simulink model "case2"  (R2024b)
settings: Solver=FixedStepAuto  StartTime=0  StopTime=1  FixedStep=1e-7  RelTol=1e-3
values from neighbouring files (symbols this model uses):
  SG_D_1_D = 0.01056    [IEEE9_case_parameters.m]    (also in case1_parameters.m; case2_parameters.m; case3_parameters.m; case4_parameters.m)
  SG_D_1_EnableSaturation = 0    [IEEE9_case_parameters.m]    (also in case1_parameters.m; case2_parameters.m; case3_parameters.m; case4_parameters.m)
  SG_D_1_f0 = 60    [IEEE9_case_parameters.m]    (also in case1_parameters.m; case2_parameters.m; case3_parameters.m; case4_parameters.m)
  SG_D_1_H = 7.5    [IEEE9_case_parameters.m]    (also in case1_parameters.m; case2_parameters.m; case3_parameters.m; case4_parameters.m)
  SG_D_1_K_A = 20    [IEEE9_case_parameters.m]    (also in case1_parameters.m; case2_parameters.m; case3_parameters.m; case4_parameters.m)
  SG_D_1_K_E = 1.000000e+1    (= 10)    [IEEE9_case_parameters.m]    (also in case1_parameters.m; case2_parameters.m; case3_parameters.m; case4_parameters.m)
  SG_D_1_K_F = 2.363    [IEEE9_case_parameters.m]    (also in case1_parameters.m; case2_parameters.m; case3_parameters.m; case4_parameters.m)
  SG_D_1_K_s = 0.5    [IEEE9_case_parameters.m]    (also in case1_parameters.m = 5; case2_parameters.m = 5; case3_parameters.m = 5; case4_parameters.m = 5)
  SG_D_1_R_a = 0.001088    [IEEE9_case_parameters.m]    (also in case1_parameters.m; case2_parameters.m; case3_parameters.m; case4_parameters.m)
  SG_D_1_S_A = 1    [IEEE9_case_parameters.m]    (also in case1_parameters.m; case2_parameters.m; case3_parameters.m; case4_parameters.m)
  SG_D_1_S_B = 0.103    [IEEE9_case_parameters.m]    (also in case1_parameters.m; case2_parameters.m; case3_parameters.m; case4_parameters.m)
  SG_D_1_S_N = 10.659857    [IEEE9_case_parameters.m]    (also in case1_parameters.m; case2_parameters.m; case3_parameters.m; case4_parameters.m)
  SG_D_1_SpeedPara = 200    [IEEE9_case_parameters.m]    (also in case1_parameters.m; case2_parameters.m; case3_parameters.m; case4_parameters.m)
  SG_D_1_T_0 = 0.720173    [IEEE9_case_parameters.m]    (also in case1_parameters.m = 0.755522; case2_parameters.m = 0.808931; case3_parameters.m = 0.869402; case4_parameters.m = 0.729316)
  SG_D_1_T_1 = 0.3    [IEEE9_case_parameters.m]    (also in case1_parameters.m; case2_parameters.m; case3_parameters.m; case4_parameters.m)
  SG_D_1_T_2 = 0.05    [IEEE9_case_parameters.m]    (also in case1_parameters.m; case2_parameters.m; case3_parameters.m; case4_parameters.m)
  SG_D_1_T_3 = 0.02    [IEEE9_case_parameters.m]    (also in case1_parameters.m; case2_parameters.m; case3_parameters.m; case4_parameters.m)
  SG_D_1_T_4 = 0.005    [IEEE9_case_parameters.m]    (also in case1_parameters.m; case2_parameters.m; case3_parameters.m; case4_parameters.m)
  SG_D_1_T_A = 0.02    [IEEE9_case_parameters.m]    (also in case1_parameters.m; case2_parameters.m; case3_parameters.m; case4_parameters.m)
  SG_D_1_T_dd = 8.000000e+0    (= 8)    [IEEE9_case_parameters.m]    (also in case1_parameters.m; case2_parameters.m; case3_parameters.m; case4_parameters.m)
  SG_D_1_T_ddd = 0.04    [IEEE9_case_parameters.m]    (also in case1_parameters.m; case2_parameters.m; case3_parameters.m; case4_parameters.m)
  SG_D_1_T_E = 0.314    [IEEE9_case_parameters.m]    (also in case1_parameters.m; case2_parameters.m; case3_parameters.m; case4_parameters.m)
  SG_D_1_T_F = 0.35    [IEEE9_case_parameters.m]    (also in case1_parameters.m; case2_parameters.m; case3_parameters.m; case4_parameters.m)
  SG_D_1_T_qd = 0.8    [IEEE9_case_parameters.m]    (also in case1_parameters.m; case2_parameters.m; case3_parameters.m; case4_parameters.m)
  SG_D_1_T_qdd = 0.02    [IEEE9_case_parameters.m]    (also in case1_parameters.m; case2_parameters.m; case3_parameters.m; case4_parameters.m)
  SG_D_1_T_speed = 0.1    [IEEE9_case_parameters.m]    (also in case1_parameters.m = 200; case2_parameters.m = 200; case3_parameters.m = 200; case4_parameters.m = 200)
  SG_D_1_T_w = 0.5    [IEEE9_case_parameters.m]    (also in case1_parameters.m; case2_parameters.m; case3_parameters.m; case4_parameters.m)
  SG_D_1_V_ref = 1.990276    [IEEE9_case_parameters.m]    (also in case1_parameters.m = 2.042296; case2_parameters.m = 2.051388; case3_parameters.m = 2.089584; case4_parameters.m = 2.01845)
  SG_D_1_w_ref = 376.991118    [IEEE9_case_parameters.m]    (also in case1_parameters.m; case2_parameters.m; case3_parameters.m; case4_parameters.m)
  SG_D_1_wb = 6.000000e+1    (= 60)    [IEEE9_case_parameters.m]    (also in case1_parameters.m; case2_parameters.m; case3_parameters.m; case4_parameters.m)
  SG_D_1_x_d = 1.9    [IEEE9_case_parameters.m]    (also in case1_parameters.m; case2_parameters.m; case3_parameters.m; case4_parameters.m)
  SG_D_1_x_dd = 0.302    [IEEE9_case_parameters.m]    (also in case1_parameters.m; case2_parameters.m; case3_parameters.m; case4_parameters.m)
  SG_D_1_x_ddd = 0.204    [IEEE9_case_parameters.m]    (also in case1_parameters.m; case2_parameters.m; case3_parameters.m; case4_parameters.m)
  SG_D_1_x_l = 0.05    [IEEE9_case_parameters.m]    (also in case1_parameters.m; case2_parameters.m; case3_parameters.m; case4_parameters.m)
  SG_D_1_x_q = 1.3    [IEEE9_case_parameters.m]    (also in case1_parameters.m; case2_parameters.m; case3_parameters.m; case4_parameters.m)
  SG_D_1_x_qd = 0.5    [IEEE9_case_parameters.m]    (also in case1_parameters.m; case2_parameters.m; case3_parameters.m; case4_parameters.m)
  SG_D_1_x_qdd = 0.3    [IEEE9_case_parameters.m]    (also in case1_parameters.m; case2_parameters.m; case3_parameters.m; case4_parameters.m)
  SG_D_2_D = 0.02    [IEEE9_case_parameters.m]    (also in case1_parameters.m; case2_parameters.m; case3_parameters.m; case4_parameters.m)
  SG_D_2_EnableSaturation = 0    [IEEE9_case_parameters.m]    (also in case1_parameters.m; case2_parameters.m; case3_parameters.m; case4_parameters.m)
  SG_D_2_f0 = 60    [IEEE9_case_parameters.m]    (also in case1_parameters.m; case2_parameters.m; case3_parameters.m; case4_parameters.m)
  SG_D_2_H = 8.000000e+0    (= 8)    [IEEE9_case_parameters.m]    (also in case1_parameters.m; case2_parameters.m; case3_parameters.m; case4_parameters.m)
  SG_D_2_K_A = 20    [IEEE9_case_parameters.m]    (also in case1_parameters.m; case2_parameters.m; case3_parameters.m; case4_parameters.m)
  SG_D_2_K_E = 1.000000e+1    (= 10)    [IEEE9_case_parameters.m]    (also in case1_parameters.m; case2_parameters.m; case3_parameters.m; case4_parameters.m)
  SG_D_2_K_F = 2.363    [IEEE9_case_parameters.m]    (also in case1_parameters.m; case2_parameters.m; case3_parameters.m; case4_parameters.m)
  SG_D_2_K_s = 0.5    [IEEE9_case_parameters.m]    (also in case1_parameters.m = 4; case2_parameters.m = 4; case3_parameters.m = 4; case4_parameters.m = 4)
  SG_D_2_R_a = 0.001088    [IEEE9_case_parameters.m]    (also in case1_parameters.m; case2_parameters.m; case3_parameters.m; case4_parameters.m)
  SG_D_2_S_A = 1    [IEEE9_case_parameters.m]    (also in case1_parameters.m; case2_parameters.m; case3_parameters.m; case4_parameters.m)
  SG_D_2_S_B = 0.103    [IEEE9_case_parameters.m]    (also in case1_parameters.m; case2_parameters.m; case3_parameters.m; case4_parameters.m)
  SG_D_2_S_N = 10.659857    [IEEE9_case_parameters.m]    (also in case1_parameters.m; case2_parameters.m; case3_parameters.m; case4_parameters.m)
  SG_D_2_SpeedPara = 200    [IEEE9_case_parameters.m]    (also in case1_parameters.m; case2_parameters.m; case3_parameters.m; case4_parameters.m)
  SG_D_2_T_0 = 1.632913    [IEEE9_case_parameters.m]    (also in case1_parameters.m = 1.632925; case2_parameters.m = 1.632915; case3_parameters.m = 1.632914; case4_parameters.m = 1.632927)
  SG_D_2_T_1 = 0.2    [IEEE9_case_parameters.m]    (also in case1_parameters.m; case2_parameters.m; case3_parameters.m; case4_parameters.m)
  SG_D_2_T_2 = 0.05    [IEEE9_case_parameters.m]    (also in case1_parameters.m; case2_parameters.m; case3_parameters.m; case4_parameters.m)
  SG_D_2_T_3 = 0.02    [IEEE9_case_parameters.m]    (also in case1_parameters.m; case2_parameters.m; case3_parameters.m; case4_parameters.m)
  SG_D_2_T_4 = 0.005    [IEEE9_case_parameters.m]    (also in case1_parameters.m; case2_parameters.m; case3_parameters.m; case4_parameters.m)
  SG_D_2_T_A = 0.02    [IEEE9_case_parameters.m]    (also in case1_parameters.m; case2_parameters.m; case3_parameters.m; case4_parameters.m)
  SG_D_2_T_dd = 7.9    [IEEE9_case_parameters.m]    (also in case1_parameters.m; case2_parameters.m; case3_parameters.m; case4_parameters.m)
  SG_D_2_T_ddd = 0.04    [IEEE9_case_parameters.m]    (also in case1_parameters.m; case2_parameters.m; case3_parameters.m; case4_parameters.m)
  SG_D_2_T_E = 0.314    [IEEE9_case_parameters.m]    (also in case1_parameters.m; case2_parameters.m; case3_parameters.m; case4_parameters.m)
  SG_D_2_T_F = 0.35    [IEEE9_case_parameters.m]    (also in case1_parameters.m; case2_parameters.m; case3_parameters.m; case4_parameters.m)
  SG_D_2_T_qd = 0.8    [IEEE9_case_parameters.m]    (also in case1_parameters.m; case2_parameters.m; case3_parameters.m; case4_parameters.m)
  SG_D_2_T_qdd = 0.015    [IEEE9_case_parameters.m]    (also in case1_parameters.m; case2_parameters.m; case3_parameters.m; case4_parameters.m)
  SG_D_2_T_speed = 0.1    [IEEE9_case_parameters.m]    (also in case1_parameters.m = 150; case2_parameters.m = 150; case3_parameters.m = 150; case4_parameters.m = 150)
  SG_D_2_T_w = 0.35    [IEEE9_case_parameters.m]    (also in case1_parameters.m; case2_parameters.m; case3_parameters.m; case4_parameters.m)
  SG_D_2_V_ref = 2.58547    [IEEE9_case_parameters.m]    (also in case1_parameters.m = 2.597896; case2_parameters.m = 2.587136; case3_parameters.m = 2.586042; case4_parameters.m = 2.599679)
  SG_D_2_w_ref = 376.991118    [IEEE9_case_parameters.m]    (also in case1_parameters.m; case2_parameters.m; case3_parameters.m; case4_parameters.m)
  SG_D_2_wb = 6.000000e+1    (= 60)    [IEEE9_case_parameters.m]    (also in case1_parameters.m; case2_parameters.m; case3_parameters.m; case4_parameters.m)
  SG_D_2_x_d = 1.8    [IEEE9_case_parameters.m]    (also in case1_parameters.m; case2_parameters.m; case3_parameters.m; case4_parameters.m)
  SG_D_2_x_dd = 0.302    [IEEE9_case_parameters.m]    (also in case1_parameters.m; case2_parameters.m; case3_parameters.m; case4_parameters.m)
  SG_D_2_x_ddd = 0.204    [IEEE9_case_parameters.m]    (also in case1_parameters.m; case2_parameters.m; case3_parameters.m; case4_parameters.m)
  SG_D_2_x_l = 0.05    [IEEE9_case_parameters.m]    (also in case1_parameters.m; case2_parameters.m; case3_parameters.m; case4_parameters.m)
  SG_D_2_x_q = 1.25    [IEEE9_case_parameters.m]    (also in case1_parameters.m; case2_parameters.m; case3_parameters.m; case4_parameters.m)
  SG_D_2_x_qd = 0.5    [IEEE9_case_parameters.m]    (also in case1_parameters.m; case2_parameters.m; case3_parameters.m; case4_parameters.m)
  SG_D_2_x_qdd = 0.3    [IEEE9_case_parameters.m]    (also in case1_parameters.m; case2_parameters.m; case3_parameters.m; case4_parameters.m)
  SG_D_3_D = 0.02    [IEEE9_case_parameters.m]    (also in case1_parameters.m; case2_parameters.m; case3_parameters.m; case4_parameters.m)
  SG_D_3_EnableSaturation = 0    [IEEE9_case_parameters.m]    (also in case1_parameters.m; case2_parameters.m; case3_parameters.m; case4_parameters.m)
  SG_D_3_f0 = 60    [IEEE9_case_parameters.m]    (also in case1_parameters.m; case2_parameters.m; case3_parameters.m; case4_parameters.m)
  SG_D_3_H = 7.7    [IEEE9_case_parameters.m]    (also in case1_parameters.m; case2_parameters.m; case3_parameters.m; case4_parameters.m)
  SG_D_3_K_A = 20    [IEEE9_case_parameters.m]    (also in case1_parameters.m; case2_parameters.m; case3_parameters.m; case4_parameters.m)
  SG_D_3_K_E = 1.000000e+1    (= 10)    [IEEE9_case_parameters.m]    (also in case1_parameters.m; case2_parameters.m; case3_parameters.m; case4_parameters.m)
  SG_D_3_K_F = 2.363    [IEEE9_case_parameters.m]    (also in case1_parameters.m; case2_parameters.m; case3_parameters.m; case4_parameters.m)
  SG_D_3_K_s = 0.2    [IEEE9_case_parameters.m]    (also in case1_parameters.m = 2; case2_parameters.m = 2; case3_parameters.m = 2; case4_parameters.m = 2)
  SG_D_3_R_a = 0.001088    [IEEE9_case_parameters.m]    (also in case1_parameters.m; case2_parameters.m; case3_parameters.m; case4_parameters.m)
  SG_D_3_S_A = 1    [IEEE9_case_parameters.m]    (also in case1_parameters.m; case2_parameters.m; case3_parameters.m; case4_parameters.m)
  SG_D_3_S_B = 0.103    [IEEE9_case_parameters.m]    (also in case1_parameters.m; case2_parameters.m; case3_parameters.m; case4_parameters.m)
  SG_D_3_S_N = 10.659857    [IEEE9_case_parameters.m]    (also in case1_parameters.m; case2_parameters.m; case3_parameters.m; case4_parameters.m)
  SG_D_3_SpeedPara = 200    [IEEE9_case_parameters.m]    (also in case1_parameters.m; case2_parameters.m; case3_parameters.m; case4_parameters.m)
  SG_D_3_T_0 = 0.850788    [IEEE9_case_parameters.m]    (also in case1_parameters.m = 0.850786; case2_parameters.m = 0.850787; case3_parameters.m; case4_parameters.m = 0.850786)
  SG_D_3_T_1 = 0.2    [IEEE9_case_parameters.m]    (also in case1_parameters.m; case2_parameters.m; case3_parameters.m; case4_parameters.m)
  SG_D_3_T_2 = 0.05    [IEEE9_case_parameters.m]    (also in case1_parameters.m; case2_parameters.m; case3_parameters.m; case4_parameters.m)
  SG_D_3_T_3 = 0.02    [IEEE9_case_parameters.m]    (also in case1_parameters.m; case2_parameters.m; case3_parameters.m; case4_parameters.m)
  SG_D_3_T_4 = 0.005    [IEEE9_case_parameters.m]    (also in case1_parameters.m; case2_parameters.m; case3_parameters.m; case4_parameters.m)
  SG_D_3_T_A = 0.02    [IEEE9_case_parameters.m]    (also in case1_parameters.m; case2_parameters.m; case3_parameters.m; case4_parameters.m)
  SG_D_3_T_dd = 8.1    [IEEE9_case_parameters.m]    (also in case1_parameters.m; case2_parameters.m; case3_parameters.m; case4_parameters.m)
  SG_D_3_T_ddd = 0.04    [IEEE9_case_parameters.m]    (also in case1_parameters.m; case2_parameters.m; case3_parameters.m; case4_parameters.m)
  SG_D_3_T_E = 0.314    [IEEE9_case_parameters.m]    (also in case1_parameters.m; case2_parameters.m; case3_parameters.m; case4_parameters.m)
  SG_D_3_T_F = 0.35    [IEEE9_case_parameters.m]    (also in case1_parameters.m; case2_parameters.m; case3_parameters.m; case4_parameters.m)
  SG_D_3_T_qd = 0.8    [IEEE9_case_parameters.m]    (also in case1_parameters.m; case2_parameters.m; case3_parameters.m; case4_parameters.m)
  SG_D_3_T_qdd = 0.015    [IEEE9_case_parameters.m]    (also in case1_parameters.m; case2_parameters.m; case3_parameters.m; case4_parameters.m)
  SG_D_3_T_speed = 0.1    [IEEE9_case_parameters.m]    (also in case1_parameters.m = 180; case2_parameters.m = 180; case3_parameters.m = 180; case4_parameters.m = 180)
  SG_D_3_T_w = 0.4    [IEEE9_case_parameters.m]    (also in case1_parameters.m; case2_parameters.m; case3_parameters.m; case4_parameters.m)
  SG_D_3_V_ref = 1.892727    [IEEE9_case_parameters.m]    (also in case1_parameters.m = 1.906439; case2_parameters.m = 1.895535; case3_parameters.m = 1.892105; case4_parameters.m = 1.906598)
  SG_D_3_w_ref = 376.991118    [IEEE9_case_parameters.m]    (also in case1_parameters.m; case2_parameters.m; case3_parameters.m; case4_parameters.m)
  SG_D_3_wb = 6.000000e+1    (= 60)    [IEEE9_case_parameters.m]    (also in case1_parameters.m; case2_parameters.m; case3_parameters.m; case4_parameters.m)
  SG_D_3_x_d = 1.85    [IEEE9_case_parameters.m]    (also in case1_parameters.m; case2_parameters.m; case3_parameters.m; case4_parameters.m)
  SG_D_3_x_dd = 0.302    [IEEE9_case_parameters.m]    (also in case1_parameters.m; case2_parameters.m; case3_parameters.m; case4_parameters.m)
  SG_D_3_x_ddd = 0.204    [IEEE9_case_parameters.m]    (also in case1_parameters.m; case2_parameters.m; case3_parameters.m; case4_parameters.m)
  SG_D_3_x_l = 0.05    [IEEE9_case_parameters.m]    (also in case1_parameters.m; case2_parameters.m; case3_parameters.m; case4_parameters.m)
  SG_D_3_x_q = 1.2    [IEEE9_case_parameters.m]    (also in case1_parameters.m; case2_parameters.m; case3_parameters.m; case4_parameters.m)
  SG_D_3_x_qd = 0.5    [IEEE9_case_parameters.m]    (also in case1_parameters.m; case2_parameters.m; case3_parameters.m; case4_parameters.m)
  SG_D_3_x_qdd = 0.3    [IEEE9_case_parameters.m]    (also in case1_parameters.m; case2_parameters.m; case3_parameters.m; case4_parameters.m)
(part 3 of 12)

== system case2/AC_1/d_id_load_7_block ==
  note: d_id_load_7 in case2
      | $376.991118430775\,\mathrm{iq}_{\mathrm{load},7}-1094.41926714385\,\mathrm{id}_{\mathrm{load},7}+1297.48703148083\,\mathrm{vd}_{\mathrm{bus},7}$
      | Automatically generated on 2025-10-31 18:56:46 .
  State_id_load_7_50270 : Inport
  State_iq_load_7_f0642 : Inport  Port=2
  State_vd_bus_7_8233e : Inport  Port=3
  Add_35670 : Sum
  Add_ebaa6 : Sum
  Constant_-1094.41926714385_6f1bd : Constant  Value=-1094.41926714385
  Constant_1297.48703148083_7e1ab : Constant  Value=1297.48703148083
  Constant_376.991118430775_2a44c : Constant  Value=376.991118430775
  Product_56fc3 : Product
  Product_c3dd4 : Product
  Product_fbb26 : Product
  Blockout_d_id_load_7_5a75a : Outport
  wires:
  Constant_-1094.41926714385_6f1bd/1 -> Product_56fc3/1
  Product_fbb26/1 -> Add_ebaa6/2
  State_id_load_7_50270/1 -> Product_56fc3/2
  Constant_376.991118430775_2a44c/1 -> Product_fbb26/1
  Product_56fc3/1 -> Add_ebaa6/1
  State_iq_load_7_f0642/1 -> Product_fbb26/2
  Constant_1297.48703148083_7e1ab/1 -> Product_c3dd4/1
  State_vd_bus_7_8233e/1 -> Product_c3dd4/2
  Add_ebaa6/1 -> Add_35670/1
  Product_c3dd4/1 -> Add_35670/2
  Add_35670/1 -> Blockout_d_id_load_7_5a75a/1

== system case2/AC_1/d_id_load_9_block ==
  note: d_id_load_9 in case2
      | $376.991118430775\,\mathrm{iq}_{\mathrm{load},9}-957.616858632595\,\mathrm{id}_{\mathrm{load},9}+1549.09705910486\,\mathrm{vd}_{\mathrm{bus},9}$
      | Automatically generated on 2025-10-31 18:56:48 .
  State_id_load_9_4df15 : Inport
  State_iq_load_9_81910 : Inport  Port=2
  State_vd_bus_9_f0529 : Inport  Port=3
  Add_4a38f : Sum
  Add_6215e : Sum
  Constant_-957.616858632595_0e708 : Constant  Value=-957.616858632595
  Constant_1549.09705910486_dd334 : Constant  Value=1549.09705910486
  Constant_376.991118430775_a5bfc : Constant  Value=376.991118430775
  Product_47c36 : Product
  Product_61caa : Product
  Product_d12cf : Product
  Blockout_d_id_load_9_4d2d3 : Outport
  wires:
  Constant_-957.616858632595_0e708/1 -> Product_47c36/1
  Product_61caa/1 -> Add_4a38f/2
  State_id_load_9_4df15/1 -> Product_47c36/2
  Constant_376.991118430775_a5bfc/1 -> Product_61caa/1
  Product_47c36/1 -> Add_4a38f/1
  State_iq_load_9_81910/1 -> Product_61caa/2
  Constant_1549.09705910486_dd334/1 -> Product_d12cf/1
  State_vd_bus_9_f0529/1 -> Product_d12cf/2
  Add_4a38f/1 -> Add_6215e/1
  Product_d12cf/1 -> Add_6215e/2
  Add_6215e/1 -> Blockout_d_id_load_9_4d2d3/1

== system case2/AC_1/d_iq_line_1_4_block ==
  note: d_iq_line_1_4 in case2
      | $6679.98156752849\,\mathrm{vq}_{\mathrm{bus},1}-376.991118430775\,\mathrm{id}_{\mathrm{line},1,4}-6679.98156752849\,\mathrm{vq}_{\mathrm{bus},4}$
      | Automatically generated on 2025-10-31 18:56:51 .
  State_id_line_1_4_24448 : Inport
  State_vq_bus_1_ed792 : Inport  Port=2
  State_vq_bus_4_1e5cd : Inport  Port=3
  Add_3527d : Sum
  Constant_-376.991118430775_76f6f : Constant  Value=-376.991118430775
  Constant_6679.98156752849_7c1df : Constant  Value=6679.98156752849
  Constant_6679.98156752849_cc398 : Constant  Value=6679.98156752849
  Product_18bbc : Product
  Product_34f2a : Product
  Product_e2593 : Product
  Subtract_9104e : Sum  Inputs=+-
  Blockout_d_iq_line_1_4_76297 : Outport
  wires:
  Constant_-376.991118430775_76f6f/1 -> Product_34f2a/1
  Product_18bbc/1 -> Add_3527d/2
  State_id_line_1_4_24448/1 -> Product_34f2a/2
  Constant_6679.98156752849_cc398/1 -> Product_18bbc/1
  Product_34f2a/1 -> Add_3527d/1
  Subtract_9104e/1 -> Blockout_d_iq_line_1_4_76297/1
  State_vq_bus_1_ed792/1 -> Product_18bbc/2
  Constant_6679.98156752849_7c1df/1 -> Product_e2593/1
  State_vq_bus_4_1e5cd/1 -> Product_e2593/2
  Add_3527d/1 -> Subtract_9104e/1
  Product_e2593/1 -> Subtract_9104e/2

== system case2/AC_1/d_iq_line_3_6_block ==
  note: d_iq_line_3_6 in case2
      | $6565.98870801435\,\mathrm{vq}_{\mathrm{bus},3}-376.991118430775\,\mathrm{id}_{\mathrm{line},3,6}-6565.98870801435\,\mathrm{vq}_{\mathrm{bus},6}$
      | Automatically generated on 2025-10-31 18:56:58 .
  State_id_line_3_6_9bf1f : Inport
  State_vq_bus_3_40690 : Inport  Port=2
  State_vq_bus_6_81b3c : Inport  Port=3
  Add_c3399 : Sum
  Constant_-376.991118430775_25eb7 : Constant  Value=-376.991118430775
  Constant_6565.98870801435_66d03 : Constant  Value=6565.98870801435
  Constant_6565.98870801435_ebb22 : Constant  Value=6565.98870801435
  Product_032d5 : Product
  Product_dcaed : Product
  Product_f987d : Product
  Subtract_72c38 : Sum  Inputs=+-
  Blockout_d_iq_line_3_6_4acdf : Outport
  wires:
  Constant_-376.991118430775_25eb7/1 -> Product_dcaed/1
  Product_032d5/1 -> Add_c3399/2
  State_id_line_3_6_9bf1f/1 -> Product_dcaed/2
  Constant_6565.98870801435_66d03/1 -> Product_032d5/1
  Product_dcaed/1 -> Add_c3399/1
  State_vq_bus_3_40690/1 -> Product_032d5/2
  Constant_6565.98870801435_ebb22/1 -> Product_f987d/1
  State_vq_bus_6_81b3c/1 -> Product_f987d/2
  Add_c3399/1 -> Subtract_72c38/1
  Product_f987d/1 -> Subtract_72c38/2
  Subtract_72c38/1 -> Blockout_d_iq_line_3_6_4acdf/1

== system case2/AC_1/d_iq_line_4_5_block ==
  note: d_iq_line_4_5 in case2
      | $4182.24932923523\,\mathrm{vq}_{\mathrm{bus},4}-67.4428209618997\,\mathrm{iq}_{\mathrm{line},4,5}-376.991118430775\,\mathrm{id}_{\mathrm{line},4,5}-4182.24932923523\,\mathrm{vq}_{\mathrm{bus},5}$
      | Automatically generated on 2025-10-31 18:56:53 .
  State_id_line_4_5_89819 : Inport
  State_iq_line_4_5_9f9c8 : Inport  Port=2
  State_vq_bus_4_4222a : Inport  Port=3
  State_vq_bus_5_9a267 : Inport  Port=4
  Add_fb21f : Sum
  Constant_-376.991118430775_b2d1d : Constant  Value=-376.991118430775
  Constant_4182.24932923523_75ca3 : Constant  Value=4182.24932923523
  Constant_4182.24932923523_77eb7 : Constant  Value=4182.24932923523
  Constant_67.4428209618997_81c5e : Constant  Value=67.4428209618997
  Product_6120d : Product
  Product_8de50 : Product
  Product_b7ec1 : Product
  Product_fd50d : Product
  Subtract_cacc3 : Sum  Inputs=+-
  Subtract_ff94e : Sum  Inputs=+-
  Blockout_d_iq_line_4_5_94582 : Outport
  wires:
  Constant_-376.991118430775_b2d1d/1 -> Product_b7ec1/1
  Constant_67.4428209618997_81c5e/1 -> Product_fd50d/1
  State_id_line_4_5_89819/1 -> Product_b7ec1/2
  State_iq_line_4_5_9f9c8/1 -> Product_fd50d/2
  Product_b7ec1/1 -> Subtract_cacc3/1
  Constant_4182.24932923523_77eb7/1 -> Product_8de50/1
  Product_fd50d/1 -> Subtract_cacc3/2
  State_vq_bus_4_4222a/1 -> Product_8de50/2
  Subtract_cacc3/1 -> Add_fb21f/1
  Product_8de50/1 -> Add_fb21f/2
  Constant_4182.24932923523_75ca3/1 -> Product_6120d/1
  State_vq_bus_5_9a267/1 -> Product_6120d/2
  Add_fb21f/1 -> Subtract_ff94e/1
  Product_6120d/1 -> Subtract_ff94e/2
  Subtract_ff94e/1 -> Blockout_d_iq_line_4_5_94582/1

== system case2/AC_1/d_iq_line_5_6_block ==
  note: d_iq_line_5_6 in case2
      | $2263.33493111553\,\mathrm{vq}_{\mathrm{bus},5}-83.7317791042547\,\mathrm{iq}_{\mathrm{line},5,6}-376.991118430775\,\mathrm{id}_{\mathrm{line},5,6}-2263.33493111553\,\mathrm{vq}_{\mathrm{bus},6}$
      | Automatically generated on 2025-10-31 18:56:56 .
  State_id_line_5_6_a16ef : Inport
  State_iq_line_5_6_db011 : Inport  Port=2
  State_vq_bus_5_e8aa3 : Inport  Port=3
  State_vq_bus_6_0b890 : Inport  Port=4
  Add_30d38 : Sum
  Constant_-376.991118430775_87ab9 : Constant  Value=-376.991118430775
  Constant_2263.33493111553_90c28 : Constant  Value=2263.33493111553
  Constant_2263.33493111553_e9e16 : Constant  Value=2263.33493111553
  Constant_83.7317791042547_646d2 : Constant  Value=83.7317791042547
  Product_1494f : Product
  Product_150c3 : Product
  Product_6eaa3 : Product
  Product_bdba7 : Product
  Subtract_05080 : Sum  Inputs=+-
  Subtract_f4bec : Sum  Inputs=+-
  Blockout_d_iq_line_5_6_4f412 : Outport
  wires:
  Constant_-376.991118430775_87ab9/1 -> Product_150c3/1
  Constant_83.7317791042547_646d2/1 -> Product_bdba7/1
  Subtract_f4bec/1 -> Blockout_d_iq_line_5_6_4f412/1
  State_id_line_5_6_a16ef/1 -> Product_150c3/2
  State_iq_line_5_6_db011/1 -> Product_bdba7/2
  Product_150c3/1 -> Subtract_05080/1
  Constant_2263.33493111553_e9e16/1 -> Product_6eaa3/1
  Product_bdba7/1 -> Subtract_05080/2
  Product_1494f/1 -> Subtract_f4bec/2
  State_vq_bus_5_e8aa3/1 -> Product_6eaa3/2
  Subtract_05080/1 -> Add_30d38/1
  Product_6eaa3/1 -> Add_30d38/2
  Constant_2263.33493111553_90c28/1 -> Product_1494f/1
  State_vq_bus_6_0b890/1 -> Product_1494f/2
  Add_30d38/1 -> Subtract_f4bec/1

== system case2/AC_1/d_iq_line_6_7_block ==
  note: d_iq_line_6_7 in case2
      | $3817.13232430199\,\mathrm{vq}_{\mathrm{bus},6}-43.0884689478804\,\mathrm{iq}_{\mathrm{line},6,7}-376.991118430775\,\mathrm{id}_{\mathrm{line},6,7}-3817.13232430199\,\mathrm{vq}_{\mathrm{bus},7}$
      | Automatically generated on 2025-10-31 18:57:00 .
  State_id_line_6_7_327c8 : Inport
  State_iq_line_6_7_06b4f : Inport  Port=2
  State_vq_bus_6_1b0a3 : Inport  Port=3
  State_vq_bus_7_35686 : Inport  Port=4
  Add_9c57b : Sum
  Constant_-376.991118430775_7dabf : Constant  Value=-376.991118430775
  Constant_3817.13232430199_4df34 : Constant  Value=3817.13232430199
  Constant_3817.13232430199_5ffb2 : Constant  Value=3817.13232430199
  Constant_43.0884689478804_2aee9 : Constant  Value=43.0884689478804
  Product_3ba1a : Product
  Product_7cc3e : Product
  Product_9e46b : Product
  Product_cb79b : Product
  Subtract_173ef : Sum  Inputs=+-
  Subtract_6e80c : Sum  Inputs=+-
  Blockout_d_iq_line_6_7_4ed8f : Outport
  wires:
  Constant_-376.991118430775_7dabf/1 -> Product_cb79b/1
  Constant_43.0884689478804_2aee9/1 -> Product_7cc3e/1
  State_id_line_6_7_327c8/1 -> Product_cb79b/2
  State_iq_line_6_7_06b4f/1 -> Product_7cc3e/2
  Product_cb79b/1 -> Subtract_173ef/1
  Constant_3817.13232430199_4df34/1 -> Product_3ba1a/1
  Product_7cc3e/1 -> Subtract_173ef/2
  State_vq_bus_6_1b0a3/1 -> Product_3ba1a/2
  Subtract_173ef/1 -> Add_9c57b/1
  Product_3ba1a/1 -> Add_9c57b/2
  Constant_3817.13232430199_5ffb2/1 -> Product_9e46b/1
  State_vq_bus_7_35686/1 -> Product_9e46b/2
  Add_9c57b/1 -> Subtract_6e80c/1
  Product_9e46b/1 -> Subtract_6e80c/2
  Subtract_6e80c/1 -> Blockout_d_iq_line_6_7_4ed8f/1

== system case2/AC_1/d_iq_line_7_8_block ==
  note: d_iq_line_7_8 in case2
      | $5343.98525402279\,\mathrm{vq}_{\mathrm{bus},7}-43.0884689478804\,\mathrm{iq}_{\mathrm{line},7,8}-376.991118430775\,\mathrm{id}_{\mathrm{line},7,8}-5343.98525402279\,\mathrm{vq}_{\mathrm{bus},8}$
      | Automatically generated on 2025-10-31 18:57:03 .
  State_id_line_7_8_f0710 : Inport
  State_iq_line_7_8_8dc14 : Inport  Port=2
  State_vq_bus_7_5bef0 : Inport  Port=3
  State_vq_bus_8_9183e : Inport  Port=4
  Add_6dfed : Sum
  Constant_-376.991118430775_c3f2d : Constant  Value=-376.991118430775
  Constant_43.0884689478804_088c2 : Constant  Value=43.0884689478804
  Constant_5343.98525402279_0400e : Constant  Value=5343.98525402279
  Constant_5343.98525402279_7ce17 : Constant  Value=5343.98525402279
  Product_58f5d : Product
  Product_736cb : Product
  Product_a150e : Product
  Product_dc7ab : Product
  Subtract_a0714 : Sum  Inputs=+-
  Subtract_b14af : Sum  Inputs=+-
  Blockout_d_iq_line_7_8_9efcd : Outport
  wires:
  Constant_-376.991118430775_c3f2d/1 -> Product_736cb/1
  Constant_43.0884689478804_088c2/1 -> Product_dc7ab/1
  State_id_line_7_8_f0710/1 -> Product_736cb/2
  State_iq_line_7_8_8dc14/1 -> Product_dc7ab/2
  Product_736cb/1 -> Subtract_b14af/1
  Constant_5343.98525402279_0400e/1 -> Product_a150e/1
  Product_dc7ab/1 -> Subtract_b14af/2
  State_vq_bus_7_5bef0/1 -> Product_a150e/2
  Subtract_b14af/1 -> Add_6dfed/1
  Product_a150e/1 -> Add_6dfed/2
  Constant_5343.98525402279_7ce17/1 -> Product_58f5d/1
  State_vq_bus_8_9183e/1 -> Product_58f5d/2
  Add_6dfed/1 -> Subtract_a0714/1
  Product_58f5d/1 -> Subtract_a0714/2
  Subtract_a0714/1 -> Blockout_d_iq_line_7_8_9efcd/1

== system case2/AC_1/d_iq_line_8_2_block ==
  note: d_iq_line_8_2 in case2
      | $6156.27101263426\,\mathrm{vq}_{\mathrm{bus},8}-6156.27101263426\,\mathrm{vq}_{\mathrm{bus},2}-376.991118430775\,\mathrm{id}_{\mathrm{line},8,2}$
      | Automatically generated on 2025-10-31 18:57:05 .
  State_id_line_8_2_ae494 : Inport
  State_vq_bus_2_b36b0 : Inport  Port=2
  State_vq_bus_8_91184 : Inport  Port=3
  Add_fc739 : Sum
  Constant_-376.991118430775_3c79b : Constant  Value=-376.991118430775
  Constant_6156.27101263426_6950f : Constant  Value=6156.27101263426
  Constant_6156.27101263426_bcf89 : Constant  Value=6156.27101263426
  Product_07cb9 : Product
  Product_09a07 : Product
  Product_cdc7b : Product
  Subtract_23355 : Sum  Inputs=+-
  Blockout_d_iq_line_8_2_96b77 : Outport
  wires:
  Constant_-376.991118430775_3c79b/1 -> Product_07cb9/1
  Product_cdc7b/1 -> Subtract_23355/2
  State_id_line_8_2_ae494/1 -> Product_07cb9/2
  Constant_6156.27101263426_bcf89/1 -> Product_cdc7b/1
  Product_07cb9/1 -> Subtract_23355/1
  State_vq_bus_2_b36b0/1 -> Product_cdc7b/2
  Constant_6156.27101263426_6950f/1 -> Product_09a07/1
  State_vq_bus_8_91184/1 -> Product_09a07/2
  Subtract_23355/1 -> Add_fc739/1
  Product_09a07/1 -> Add_fc739/2
  Add_fc739/1 -> Blockout_d_iq_line_8_2_96b77/1

== system case2/AC_1/d_iq_line_8_9_block ==
  note: d_iq_line_8_9 in case2
      | $2389.85675956299\,\mathrm{vq}_{\mathrm{bus},8}-72.54353851364\,\mathrm{iq}_{\mathrm{line},8,9}-376.991118430775\,\mathrm{id}_{\mathrm{line},8,9}-2389.85675956299\,\mathrm{vq}_{\mathrm{bus},9}$
      | Automatically generated on 2025-10-31 18:57:07 .
  State_id_line_8_9_f0140 : Inport
  State_iq_line_8_9_2d182 : Inport  Port=2
  State_vq_bus_8_a2731 : Inport  Port=3
  State_vq_bus_9_ce318 : Inport  Port=4
  Add_9a949 : Sum
  Constant_-376.991118430775_5d9a2 : Constant  Value=-376.991118430775
  Constant_2389.85675956299_bfeb3 : Constant  Value=2389.85675956299
  Constant_2389.85675956299_de443 : Constant  Value=2389.85675956299
  Constant_72.54353851364_d16aa : Constant  Value=72.54353851364
  Product_3da2b : Product
  Product_6fa59 : Product
  Product_99d17 : Product
  Product_b4fa4 : Product
  Subtract_4b83b : Sum  Inputs=+-
  Subtract_93370 : Sum  Inputs=+-
  Blockout_d_iq_line_8_9_92184 : Outport
  wires:
  Constant_-376.991118430775_5d9a2/1 -> Product_b4fa4/1
  Constant_72.54353851364_d16aa/1 -> Product_99d17/1
  State_id_line_8_9_f0140/1 -> Product_b4fa4/2
  State_iq_line_8_9_2d182/1 -> Product_99d17/2
  Product_b4fa4/1 -> Subtract_93370/1
  Constant_2389.85675956299_bfeb3/1 -> Product_6fa59/1
  Product_99d17/1 -> Subtract_93370/2
  State_vq_bus_8_a2731/1 -> Product_6fa59/2
  Subtract_93370/1 -> Add_9a949/1
  Product_6fa59/1 -> Add_9a949/2
  Constant_2389.85675956299_de443/1 -> Product_3da2b/1
  Add_9a949/1 -> Subtract_4b83b/1
  State_vq_bus_9_ce318/1 -> Product_3da2b/2
  Product_3da2b/1 -> Subtract_4b83b/2
  Subtract_4b83b/1 -> Blockout_d_iq_line_8_9_92184/1

== system case2/AC_1/d_iq_line_9_4_block ==
  note: d_iq_line_9_4 in case2
      | $4526.66986223107\,\mathrm{vq}_{\mathrm{bus},9}-42.9393738996178\,\mathrm{iq}_{\mathrm{line},9,4}-4526.66986223107\,\mathrm{vq}_{\mathrm{bus},4}-376.991118430775\,\mathrm{id}_{\mathrm{line},9,4}$
      | Automatically generated on 2025-10-31 18:57:10 .
  State_id_line_9_4_54433 : Inport
  State_iq_line_9_4_bf158 : Inport  Port=2
  State_vq_bus_4_44071 : Inport  Port=3
  State_vq_bus_9_c61bf : Inport  Port=4
  Add_e7da8 : Sum
  Constant_-376.991118430775_7d32a : Constant  Value=-376.991118430775
  Constant_42.9393738996178_aa086 : Constant  Value=42.9393738996178
  Constant_4526.66986223107_08b37 : Constant  Value=4526.66986223107
  Constant_4526.66986223107_171e0 : Constant  Value=4526.66986223107
  Product_31d74 : Product
  Product_91836 : Product
  Product_9a8bb : Product
  Product_be90b : Product
  Subtract_72bed : Sum  Inputs=+-
  Subtract_820b0 : Sum  Inputs=+-
  Blockout_d_iq_line_9_4_61cd6 : Outport
  wires:
  Constant_-376.991118430775_7d32a/1 -> Product_91836/1
  Constant_42.9393738996178_aa086/1 -> Product_be90b/1
  State_id_line_9_4_54433/1 -> Product_91836/2
  State_iq_line_9_4_bf158/1 -> Product_be90b/2
  Product_91836/1 -> Subtract_72bed/1
  Constant_4526.66986223107_171e0/1 -> Product_9a8bb/1
  Product_be90b/1 -> Subtract_72bed/2
  State_vq_bus_4_44071/1 -> Product_9a8bb/2
  Subtract_72bed/1 -> Subtract_820b0/1
  Product_9a8bb/1 -> Subtract_820b0/2
  Constant_4526.66986223107_08b37/1 -> Product_31d74/1
  Add_e7da8/1 -> Blockout_d_iq_line_9_4_61cd6/1
  State_vq_bus_9_c61bf/1 -> Product_31d74/2
  Subtract_820b0/1 -> Add_e7da8/1
  Product_31d74/1 -> Add_e7da8/2

== system case2/AC_1/d_iq_load_5_block ==
  note: d_iq_load_5 in case2
      | $1237.92955189927\,\mathrm{vq}_{\mathrm{bus},5}-1149.14023057989\,\mathrm{iq}_{\mathrm{load},5}-376.991118430775\,\mathrm{id}_{\mathrm{load},5}$
      | Automatically generated on 2025-10-31 18:56:45 .
  State_id_load_5_4850d : Inport
  State_iq_load_5_1b5d6 : Inport  Port=2
  State_vq_bus_5_e375c : Inport  Port=3
  Add_d4e62 : Sum
  Constant_-376.991118430775_6b2ab : Constant  Value=-376.991118430775
  Constant_1149.14023057989_ad488 : Constant  Value=1149.14023057989
  Constant_1237.92955189927_4713c : Constant  Value=1237.92955189927
  Product_353fc : Product
  Product_6a2d2 : Product
  Product_ef552 : Product
  Subtract_70751 : Sum  Inputs=+-
  Blockout_d_iq_load_5_6b6fd : Outport
  wires:
  Constant_-376.991118430775_6b2ab/1 -> Product_ef552/1
  Product_353fc/1 -> Subtract_70751/2
  State_id_load_5_4850d/1 -> Product_ef552/2
  Constant_1149.14023057989_ad488/1 -> Product_353fc/1
  Product_ef552/1 -> Subtract_70751/1
  State_iq_load_5_1b5d6/1 -> Product_353fc/2
  Constant_1237.92955189927_4713c/1 -> Product_6a2d2/1
  State_vq_bus_5_e375c/1 -> Product_6a2d2/2
  Subtract_70751/1 -> Add_d4e62/1
  Product_6a2d2/1 -> Add_d4e62/2
  Add_d4e62/1 -> Blockout_d_iq_load_5_6b6fd/1

== system case2/AC_1/d_iq_load_7_block ==
  note: d_iq_load_7 in case2
      | $1297.48703148083\,\mathrm{vq}_{\mathrm{bus},7}-1094.41926714385\,\mathrm{iq}_{\mathrm{load},7}-376.991118430775\,\mathrm{id}_{\mathrm{load},7}$
      | Automatically generated on 2025-10-31 18:56:47 .
  State_id_load_7_916b5 : Inport
  State_iq_load_7_28c55 : Inport  Port=2
  State_vq_bus_7_90b72 : Inport  Port=3
  Add_d81a1 : Sum
  Constant_-376.991118430775_53f05 : Constant  Value=-376.991118430775
  Constant_1094.41926714385_683e1 : Constant  Value=1094.41926714385
  Constant_1297.48703148083_c2701 : Constant  Value=1297.48703148083
  Product_9b467 : Product
  Product_ddb6b : Product
  Product_eee72 : Product
  Subtract_06d53 : Sum  Inputs=+-
  Blockout_d_iq_load_7_45a74 : Outport
  wires:
  Constant_-376.991118430775_53f05/1 -> Product_eee72/1
  Product_ddb6b/1 -> Subtract_06d53/2
  State_id_load_7_916b5/1 -> Product_eee72/2
  Constant_1094.41926714385_683e1/1 -> Product_ddb6b/1
  Product_eee72/1 -> Subtract_06d53/1
  State_iq_load_7_28c55/1 -> Product_ddb6b/2
  Constant_1297.48703148083_c2701/1 -> Product_9b467/1
  State_vq_bus_7_90b72/1 -> Product_9b467/2
  Subtract_06d53/1 -> Add_d81a1/1
  Product_9b467/1 -> Add_d81a1/2
  Add_d81a1/1 -> Blockout_d_iq_load_7_45a74/1

== system case2/AC_1/d_iq_load_9_block ==
  note: d_iq_load_9 in case2
      | $1549.09705910486\,\mathrm{vq}_{\mathrm{bus},9}-957.616858632595\,\mathrm{iq}_{\mathrm{load},9}-376.991118430775\,\mathrm{id}_{\mathrm{load},9}$
      | Automatically generated on 2025-10-31 18:56:49 .
  State_id_load_9_3b2fd : Inport
  State_iq_load_9_12d39 : Inport  Port=2
  State_vq_bus_9_18995 : Inport  Port=3
  Add_c27d5 : Sum
  Constant_-376.991118430775_f7c6f : Constant  Value=-376.991118430775
  Constant_1549.09705910486_80aea : Constant  Value=1549.09705910486
  Constant_957.616858632595_c7ccd : Constant  Value=957.616858632595
  Product_75bfc : Product
  Product_8d11c : Product
  Product_d06d0 : Product
  Subtract_7f738 : Sum  Inputs=+-
  Blockout_d_iq_load_9_e3180 : Outport
  wires:
  Constant_-376.991118430775_f7c6f/1 -> Product_75bfc/1
  Product_d06d0/1 -> Subtract_7f738/2
  State_id_load_9_3b2fd/1 -> Product_75bfc/2
  Add_c27d5/1 -> Blockout_d_iq_load_9_e3180/1
  Constant_957.616858632595_c7ccd/1 -> Product_d06d0/1
  Product_8d11c/1 -> Add_c27d5/2
  Product_75bfc/1 -> Subtract_7f738/1
  State_iq_load_9_12d39/1 -> Product_d06d0/2
  Constant_1549.09705910486_80aea/1 -> Product_8d11c/1
  State_vq_bus_9_18995/1 -> Product_8d11c/2
  Subtract_7f738/1 -> Add_c27d5/1

== system case2/AC_1/d_vd_bus_1_block ==
  note: d_vd_bus_1 in case2
      | $37699111.8430775\,\mathrm{id}_{\mathrm{bus},1}+376.991118430775\,\mathrm{vq}_{\mathrm{bus},1}$
      | Automatically generated on 2025-10-31 18:56:29 .
  Alge_id_bus_1_716c4 : Inport
  State_vq_bus_1_a61e0 : Inport  Port=2
  Add_c6b30 : Sum
  Constant_376.991118430775_86ae6 : Constant  Value=376.991118430775
  Constant_37699111.8430775_41787 : Constant  Value=37699111.8430775
  Product_a7524 : Product
  Product_affa2 : Product
  Blockout_d_vd_bus_1_1c28f : Outport
  wires:
  Constant_37699111.8430775_41787/1 -> Product_a7524/1
  Product_affa2/1 -> Add_c6b30/2
  Alge_id_bus_1_716c4/1 -> Product_a7524/2
  Constant_376.991118430775_86ae6/1 -> Product_affa2/1
  State_vq_bus_1_a61e0/1 -> Product_affa2/2
  Add_c6b30/1 -> Blockout_d_vd_bus_1_1c28f/1
  Product_a7524/1 -> Add_c6b30/1

== system case2/AC_1/d_vd_bus_2_block ==
  note: d_vd_bus_2 in case2
      | $37699111.8430775\,\mathrm{id}_{\mathrm{bus},2}+376.991118430775\,\mathrm{vq}_{\mathrm{bus},2}$
      | Automatically generated on 2025-10-31 18:56:31 .
  Alge_id_bus_2_d46c7 : Inport
  State_vq_bus_2_1d16a : Inport  Port=2
  Add_795f1 : Sum
  Constant_376.991118430775_02713 : Constant  Value=376.991118430775
  Constant_37699111.8430775_01c7d : Constant  Value=37699111.8430775
  Product_dc980 : Product
  Product_dfc7d : Product
  Blockout_d_vd_bus_2_5d58d : Outport
  wires:
  Constant_37699111.8430775_01c7d/1 -> Product_dfc7d/1
  Product_dc980/1 -> Add_795f1/2
  Alge_id_bus_2_d46c7/1 -> Product_dfc7d/2
  Constant_376.991118430775_02713/1 -> Product_dc980/1
  Product_dfc7d/1 -> Add_795f1/1
  State_vq_bus_2_1d16a/1 -> Product_dc980/2
  Add_795f1/1 -> Blockout_d_vd_bus_2_5d58d/1

== system case2/AC_1/d_vd_bus_3_block ==
  note: d_vd_bus_3 in case2
      | $37699111.8430775\,\mathrm{id}_{\mathrm{bus},3}+376.991118430775\,\mathrm{vq}_{\mathrm{bus},3}$
      | Automatically generated on 2025-10-31 18:56:32 .
  Alge_id_bus_3_78d4b : Inport
  State_vq_bus_3_ecd7b : Inport  Port=2
  Add_60ccf : Sum
  Constant_376.991118430775_38798 : Constant  Value=376.991118430775
  Constant_37699111.8430775_ad31d : Constant  Value=37699111.8430775
  Product_2d66c : Product
  Product_e3b73 : Product
  Blockout_d_vd_bus_3_0aed6 : Outport
  wires:
  Constant_37699111.8430775_ad31d/1 -> Product_2d66c/1
  Product_e3b73/1 -> Add_60ccf/2
  Alge_id_bus_3_78d4b/1 -> Product_2d66c/2
  Constant_376.991118430775_38798/1 -> Product_e3b73/1
  Product_2d66c/1 -> Add_60ccf/1
  State_vq_bus_3_ecd7b/1 -> Product_e3b73/2
  Add_60ccf/1 -> Blockout_d_vd_bus_3_0aed6/1

== system case2/AC_1/d_vd_bus_4_block ==
  note: d_vd_bus_4 in case2
      | $2257.43184689087\,\mathrm{id}_{\mathrm{bus},4}+376.991118430775\,\mathrm{vq}_{\mathrm{bus},4}$
      | Automatically generated on 2025-10-31 18:56:34 .
  Alge_id_bus_4_86c66 : Inport
  State_vq_bus_4_2d336 : Inport  Port=2
  Add_d4072 : Sum
  Constant_2257.43184689087_a8c1e : Constant  Value=2257.43184689087
  Constant_376.991118430775_f4cbd : Constant  Value=376.991118430775
  Product_c34b4 : Product
  Product_d2d0e : Product
  Blockout_d_vd_bus_4_39df0 : Outport
  wires:
  Constant_2257.43184689087_a8c1e/1 -> Product_d2d0e/1
  Product_c34b4/1 -> Add_d4072/2
  Alge_id_bus_4_86c66/1 -> Product_d2d0e/2
  Constant_376.991118430775_f4cbd/1 -> Product_c34b4/1
  Product_d2d0e/1 -> Add_d4072/1
  State_vq_bus_4_2d336/1 -> Product_c34b4/2
  Add_d4072/1 -> Blockout_d_vd_bus_4_39df0/1

== system case2/AC_1/d_vd_bus_5_block ==
  note: d_vd_bus_5 in case2
      | $1461.2058853906\,\mathrm{id}_{\mathrm{bus},5}+376.991118430775\,\mathrm{vq}_{\mathrm{bus},5}$
      | Automatically generated on 2025-10-31 18:56:36 .
  Alge_id_bus_5_78beb : Inport
  State_vq_bus_5_c24a2 : Inport  Port=2
  Add_bd5e7 : Sum
  Constant_1461.2058853906_cc120 : Constant  Value=1461.2058853906
  Constant_376.991118430775_93399 : Constant  Value=376.991118430775
  Product_3022d : Product
  Product_e1042 : Product
  Blockout_d_vd_bus_5_ea476 : Outport
  wires:
  Constant_1461.2058853906_cc120/1 -> Product_3022d/1
  Product_e1042/1 -> Add_bd5e7/2
  Alge_id_bus_5_78beb/1 -> Product_3022d/2
  Constant_376.991118430775_93399/1 -> Product_e1042/1
  Product_3022d/1 -> Add_bd5e7/1
  State_vq_bus_5_c24a2/1 -> Product_e1042/2
  Add_bd5e7/1 -> Blockout_d_vd_bus_5_ea476/1

== system case2/AC_1/d_vd_bus_6_block ==
  note: d_vd_bus_6 in case2
      | $1329.77466818616\,\mathrm{id}_{\mathrm{bus},6}+376.991118430775\,\mathrm{vq}_{\mathrm{bus},6}$
      | Automatically generated on 2025-10-31 18:56:37 .
  Alge_id_bus_6_030aa : Inport
  State_vq_bus_6_ee9a7 : Inport  Port=2
  Add_e0d34 : Sum
  Constant_1329.77466818616_5aa11 : Constant  Value=1329.77466818616
  Constant_376.991118430775_e1a8a : Constant  Value=376.991118430775
  Product_0fc88 : Product
  Product_300af : Product
  Blockout_d_vd_bus_6_f68c6 : Outport
  wires:
  Constant_1329.77466818616_5aa11/1 -> Product_0fc88/1
  Product_300af/1 -> Add_e0d34/2
  Alge_id_bus_6_030aa/1 -> Product_0fc88/2
  Constant_376.991118430775_e1a8a/1 -> Product_300af/1
  Product_0fc88/1 -> Add_e0d34/1
  State_vq_bus_6_ee9a7/1 -> Product_300af/2
  Add_e0d34/1 -> Blockout_d_vd_bus_6_f68c6/1

== system case2/AC_1/d_vd_bus_7_block ==
  note: d_vd_bus_7 in case2
      | $2106.09563369148\,\mathrm{id}_{\mathrm{bus},7}+376.991118430775\,\mathrm{vq}_{\mathrm{bus},7}$
      | Automatically generated on 2025-10-31 18:56:39 .
  Alge_id_bus_7_e76ec : Inport
  State_vq_bus_7_81f66 : Inport  Port=2
  Add_2f4e5 : Sum
  Constant_2106.09563369148_ae6f4 : Constant  Value=2106.09563369148
  Constant_376.991118430775_61cd1 : Constant  Value=376.991118430775
  Product_0dd5f : Product
  Product_eb8e4 : Product
  Blockout_d_vd_bus_7_1b34a : Outport
  wires:
  Constant_2106.09563369148_ae6f4/1 -> Product_0dd5f/1
  Product_eb8e4/1 -> Add_2f4e5/2
  Alge_id_bus_7_e76ec/1 -> Product_0dd5f/2
  Constant_376.991118430775_61cd1/1 -> Product_eb8e4/1
  Product_0dd5f/1 -> Add_2f4e5/1
  State_vq_bus_7_81f66/1 -> Product_eb8e4/2
  Add_2f4e5/1 -> Blockout_d_vd_bus_7_1b34a/1

== system case2/AC_1/d_vd_bus_8_block ==
  note: d_vd_bus_8 in case2
      | $1657.10381727813\,\mathrm{id}_{\mathrm{bus},8}+376.991118430775\,\mathrm{vq}_{\mathrm{bus},8}$
      | Automatically generated on 2025-10-31 18:56:40 .
  Alge_id_bus_8_f6d08 : Inport
  State_vq_bus_8_658d5 : Inport  Port=2
  Add_d22ba : Sum
  Constant_1657.10381727813_4a88a : Constant  Value=1657.10381727813
  Constant_376.991118430775_3fed8 : Constant  Value=376.991118430775
  Product_976be : Product
  Product_a1e86 : Product
  Blockout_d_vd_bus_8_439e3 : Outport
  wires:
  Constant_1657.10381727813_4a88a/1 -> Product_a1e86/1
  Product_976be/1 -> Add_d22ba/2
  Alge_id_bus_8_f6d08/1 -> Product_a1e86/2
  Constant_376.991118430775_3fed8/1 -> Product_976be/1
  Product_a1e86/1 -> Add_d22ba/1
  State_vq_bus_8_658d5/1 -> Product_976be/2
  Add_d22ba/1 -> Blockout_d_vd_bus_8_439e3/1

== system case2/AC_1/d_vd_bus_9_block ==
  note: d_vd_bus_9 in case2
      | $1564.27849971276\,\mathrm{id}_{\mathrm{bus},9}+376.991118430775\,\mathrm{vq}_{\mathrm{bus},9}$
      | Automatically generated on 2025-10-31 18:56:42 .
  Alge_id_bus_9_3932a : Inport
  State_vq_bus_9_34de9 : Inport  Port=2
  Add_b169c : Sum
  Constant_1564.27849971276_2e4ce : Constant  Value=1564.27849971276
  Constant_376.991118430775_eb034 : Constant  Value=376.991118430775
  Product_1ab7a : Product
  Product_a4fa8 : Product
  Blockout_d_vd_bus_9_65c7e : Outport
  wires:
  Constant_1564.27849971276_2e4ce/1 -> Product_1ab7a/1
  Product_a4fa8/1 -> Add_b169c/2
  Alge_id_bus_9_3932a/1 -> Product_1ab7a/2
  Constant_376.991118430775_eb034/1 -> Product_a4fa8/1
  Product_1ab7a/1 -> Add_b169c/1
  State_vq_bus_9_34de9/1 -> Product_a4fa8/2
  Add_b169c/1 -> Blockout_d_vd_bus_9_65c7e/1

== system case2/AC_1/d_vq_bus_1_block ==
  note: d_vq_bus_1 in case2
      | $37699111.8430775\,\mathrm{iq}_{\mathrm{bus},1}-376.991118430775\,\mathrm{vd}_{\mathrm{bus},1}$
      | Automatically generated on 2025-10-31 18:56:30 .
  Alge_iq_bus_1_2119b : Inport
  State_vd_bus_1_ddfcb : Inport  Port=2
  Constant_376.991118430775_86a35 : Constant  Value=376.991118430775
  Constant_37699111.8430775_b2317 : Constant  Value=37699111.8430775
  Product_248aa : Product
  Product_92391 : Product
  Subtract_183c7 : Sum  Inputs=+-
  Blockout_d_vq_bus_1_11663 : Outport
  wires:
  Constant_37699111.8430775_b2317/1 -> Product_248aa/1
  Constant_376.991118430775_86a35/1 -> Product_92391/1
  Alge_iq_bus_1_2119b/1 -> Product_248aa/2
  State_vd_bus_1_ddfcb/1 -> Product_92391/2
  Product_248aa/1 -> Subtract_183c7/1
  Product_92391/1 -> Subtract_183c7/2
  Subtract_183c7/1 -> Blockout_d_vq_bus_1_11663/1

== system case2/AC_1/d_vq_bus_2_block ==
  note: d_vq_bus_2 in case2
      | $37699111.8430775\,\mathrm{iq}_{\mathrm{bus},2}-376.991118430775\,\mathrm{vd}_{\mathrm{bus},2}$
      | Automatically generated on 2025-10-31 18:56:32 .
  Alge_iq_bus_2_5c6d8 : Inport
  State_vd_bus_2_59719 : Inport  Port=2
  Constant_376.991118430775_0d2e0 : Constant  Value=376.991118430775
  Constant_37699111.8430775_57808 : Constant  Value=37699111.8430775
  Product_34ba1 : Product
  Product_4d340 : Product
  Subtract_1cacc : Sum  Inputs=+-
  Blockout_d_vq_bus_2_0966a : Outport
  wires:
  Constant_37699111.8430775_57808/1 -> Product_4d340/1
  Constant_376.991118430775_0d2e0/1 -> Product_34ba1/1
  Alge_iq_bus_2_5c6d8/1 -> Product_4d340/2
  State_vd_bus_2_59719/1 -> Product_34ba1/2
  Product_4d340/1 -> Subtract_1cacc/1
  Product_34ba1/1 -> Subtract_1cacc/2
  Subtract_1cacc/1 -> Blockout_d_vq_bus_2_0966a/1

== system case2/AC_1/d_vq_bus_3_block ==
  note: d_vq_bus_3 in case2
      | $37699111.8430775\,\mathrm{iq}_{\mathrm{bus},3}-376.991118430775\,\mathrm{vd}_{\mathrm{bus},3}$
      | Automatically generated on 2025-10-31 18:56:33 .
  Alge_iq_bus_3_59f2b : Inport
  State_vd_bus_3_a1107 : Inport  Port=2
  Constant_376.991118430775_3743f : Constant  Value=376.991118430775
  Constant_37699111.8430775_b4f31 : Constant  Value=37699111.8430775
  Product_7e79b : Product
  Product_bc43e : Product
  Subtract_0ae47 : Sum  Inputs=+-
  Blockout_d_vq_bus_3_e5e49 : Outport
  wires:
  Constant_37699111.8430775_b4f31/1 -> Product_7e79b/1
  Constant_376.991118430775_3743f/1 -> Product_bc43e/1
  Alge_iq_bus_3_59f2b/1 -> Product_7e79b/2
  State_vd_bus_3_a1107/1 -> Product_bc43e/2
  Product_7e79b/1 -> Subtract_0ae47/1
  Product_bc43e/1 -> Subtract_0ae47/2
  Subtract_0ae47/1 -> Blockout_d_vq_bus_3_e5e49/1

== system case2/AC_1/d_vq_bus_4_block ==
  note: d_vq_bus_4 in case2
      | $2257.43184689087\,\mathrm{iq}_{\mathrm{bus},4}-376.991118430775\,\mathrm{vd}_{\mathrm{bus},4}$
      | Automatically generated on 2025-10-31 18:56:35 .
  Alge_iq_bus_4_697f2 : Inport
  State_vd_bus_4_2d95a : Inport  Port=2
  Constant_2257.43184689087_53584 : Constant  Value=2257.43184689087
  Constant_376.991118430775_85ff9 : Constant  Value=376.991118430775
  Product_b4cf5 : Product
  Product_d0adb : Product
  Subtract_76b7e : Sum  Inputs=+-
  Blockout_d_vq_bus_4_587da : Outport
  wires:
  Constant_2257.43184689087_53584/1 -> Product_d0adb/1
  Constant_376.991118430775_85ff9/1 -> Product_b4cf5/1
  Alge_iq_bus_4_697f2/1 -> Product_d0adb/2
  State_vd_bus_4_2d95a/1 -> Product_b4cf5/2
  Product_d0adb/1 -> Subtract_76b7e/1
  Product_b4cf5/1 -> Subtract_76b7e/2
  Subtract_76b7e/1 -> Blockout_d_vq_bus_4_587da/1

== system case2/AC_1/d_vq_bus_5_block ==
  note: d_vq_bus_5 in case2
      | $1461.2058853906\,\mathrm{iq}_{\mathrm{bus},5}-376.991118430775\,\mathrm{vd}_{\mathrm{bus},5}$
      | Automatically generated on 2025-10-31 18:56:36 .
  Alge_iq_bus_5_8f4e4 : Inport
  State_vd_bus_5_3b4b0 : Inport  Port=2
  Constant_1461.2058853906_39abe : Constant  Value=1461.2058853906
  Constant_376.991118430775_aa748 : Constant  Value=376.991118430775
  Product_22ffc : Product
  Product_b9088 : Product
  Subtract_f3ae0 : Sum  Inputs=+-
  Blockout_d_vq_bus_5_9db4d : Outport
  wires:
  Constant_1461.2058853906_39abe/1 -> Product_22ffc/1
  Constant_376.991118430775_aa748/1 -> Product_b9088/1
  Alge_iq_bus_5_8f4e4/1 -> Product_22ffc/2
  State_vd_bus_5_3b4b0/1 -> Product_b9088/2
  Product_22ffc/1 -> Subtract_f3ae0/1
  Product_b9088/1 -> Subtract_f3ae0/2
  Subtract_f3ae0/1 -> Blockout_d_vq_bus_5_9db4d/1

== system case2/AC_1/d_vq_bus_6_block ==
  note: d_vq_bus_6 in case2
      | $1329.77466818616\,\mathrm{iq}_{\mathrm{bus},6}-376.991118430775\,\mathrm{vd}_{\mathrm{bus},6}$
      | Automatically generated on 2025-10-31 18:56:38 .
  Alge_iq_bus_6_8b56a : Inport
  State_vd_bus_6_e4a17 : Inport  Port=2
  Constant_1329.77466818616_13c87 : Constant  Value=1329.77466818616
  Constant_376.991118430775_44515 : Constant  Value=376.991118430775
  Product_7d564 : Product
  Product_becc9 : Product
  Subtract_edd8e : Sum  Inputs=+-
  Blockout_d_vq_bus_6_8dd8e : Outport
  wires:
  Constant_1329.77466818616_13c87/1 -> Product_7d564/1
  Constant_376.991118430775_44515/1 -> Product_becc9/1
  Alge_iq_bus_6_8b56a/1 -> Product_7d564/2
  State_vd_bus_6_e4a17/1 -> Product_becc9/2
  Product_7d564/1 -> Subtract_edd8e/1
  Product_becc9/1 -> Subtract_edd8e/2
  Subtract_edd8e/1 -> Blockout_d_vq_bus_6_8dd8e/1
